simulink model "load_flow_analysis"  (R2014b)
settings: Solver=ode45  StartTime=0.0  StopTime=10.0  RelTol=1e-3
libraries: powerlib x13
settings Model: Creator=Amr Saleh  LastModifiedBy=Amr Saleh

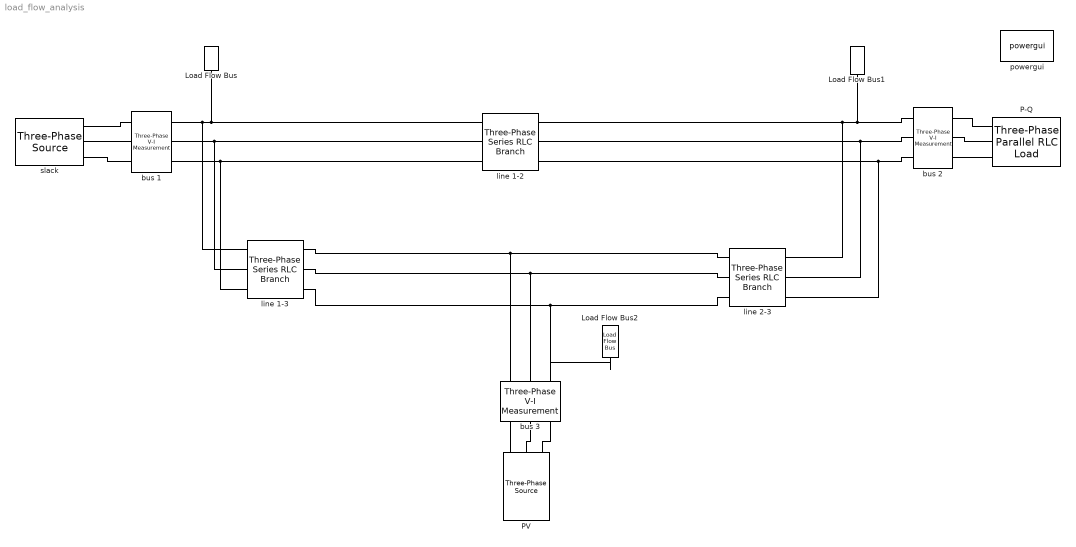
== system load_flow_analysis ==
  Load Flow Bus : powerlib/Measurements/Load Flow Bus  LConnTagsString=a  ID=BUS_1  Vbase=10e3  Vref=1.05  Vangle=0  VLF=1.05  angleLF=0
      settings: AttributesFormatString=%<ID>\n%<Vbase>V\n%<VLF>pu\n%<angleLF>deg.
  Load Flow Bus1 : powerlib/Measurements/Load Flow Bus  LConnTagsString=a  ID=BUS_2  Vbase=10e3  Vref=1  Vangle=0  VLF=0.9897  angleLF=1.546
      settings: AttributesFormatString=%<ID>\n%<Vbase>V\n%<VLF>pu\n%<angleLF>deg.
  Load Flow Bus2 : powerlib/Measurements/Load Flow Bus  LConnTagsString=a  ID=BUS_3  Vbase=10e3  Vref=1.04  Vangle=0  VLF=1.04  angleLF=3.427
      settings: AttributesFormatString=%<ID>\n%<Vbase>V\n%<VLF>pu\n%<angleLF>deg.
  P-Q : powerlib/Elements/Three-Phase Parallel RLC Load  LConnTagsString=A|B|C  Configuration=Y (grounded)  NominalVoltage=10e3  NominalFrequency=60  ActivePower=190e6  InductivePower=250e6  CapacitivePower=0  Measurements=None  LoadType=constant PQ
  PV : powerlib/Electrical Sources/Three-Phase Source  Voltage=10e3  PhaseAngle=0  Frequency=60  InternalConnection=Yg  SpecifyImpedance=off  Resistance=0.8929  Inductance=16.58e-3  ShortCircuitLevel=100e6  BaseVoltage=10e3  XRratio=7  BusType=PV  Pref=380e6  Qref=0  Qmin=-inf  Qmax=inf
  bus 1 : powerlib/Measurements/Three-Phase V-I Measurement  VoltageMeasurement=no  SetLabelV=off  LabelV=Vabc  Vpu=off  VpuLL=off  CurrentMeasurement=no  SetLabelI=off  LabelI=Iabc  Ipu=off  Pbase=100e6  Vbase=500e3  OutputType=Complex  PhasorSimulation=off  PSBequivalent=0
  bus 2 : powerlib/Measurements/Three-Phase V-I Measurement  VoltageMeasurement=no  SetLabelV=off  LabelV=Vabc  Vpu=off  VpuLL=off  CurrentMeasurement=no  SetLabelI=off  LabelI=Iabc  Ipu=off  Pbase=100e6  Vbase=500e3  OutputType=Complex  PhasorSimulation=off  PSBequivalent=0
  bus 3 : powerlib/Measurements/Three-Phase V-I Measurement  VoltageMeasurement=no  SetLabelV=off  LabelV=Vabc  Vpu=off  VpuLL=off  CurrentMeasurement=no  SetLabelI=off  LabelI=Iabc  Ipu=off  Pbase=100e6  Vbase=500e3  OutputType=Complex  PhasorSimulation=off  PSBequivalent=0
  line 1-2 : powerlib/Elements/Three-Phase Series RLC Branch  LConnTagsString=A|B|C  RConnTagsString=A|B|C  BranchType=RL  Resistance=0.02  Inductance=0.04/(2*pi*60)  Capacitance=1e-6  Measurements=None
  line 1-3 : powerlib/Elements/Three-Phase Series RLC Branch  LConnTagsString=A|B|C  RConnTagsString=A|B|C  BranchType=RL  Resistance=0.01  Inductance=0.03/(2*pi*60)  Capacitance=1e-6  Measurements=None
  line 2-3 : powerlib/Elements/Three-Phase Series RLC Branch  LConnTagsString=A|B|C  RConnTagsString=A|B|C  BranchType=RL  Resistance=0.0125  Inductance=0.025/(2*pi*60)  Capacitance=1e-6  Measurements=None
  powergui : powerlib/powergui  Priority=1  SimulationMode=Continuous  SolverType=Tustin/Backward Euler (TBE)  SampleTime=50e-6  frequency=60  SPID=off  DisableSnubberDevices=off  DisableRonSwitches=off  DisableVfSwitches=off  SwTol=0  DisplayEquations=off  Interpol=off  methode=off  Ts=100  frequencyindice=60  Pbase=100e6  ErrMax=0.0001  Iterations=50  UnitsV=kV  UnitsW=MW  FunctionMessages=off  echomessages=off  HookPort=off  EnableUseOfTLC=off  x0status=blocks  RestoreLinks=warning  ResistiveCurrentMeasurement=off  Frange=[0:2:500]  Ylog=off  Xlog=on  ShowGrid=off  save=off  variable=ZData  structure=0  ZoomFFT=off  StartTime=0.0  cycles=1  DisplayStyle=1  fundamental=60  FreqAxis=off  MaxFrequency=1000  frequencyindicesteady=1  RmsSteady=1  display=off
  slack : powerlib/Electrical Sources/Three-Phase Source  Voltage=10e3  PhaseAngle=0  Frequency=60  InternalConnection=Yg  SpecifyImpedance=off  Resistance=0.8929  Inductance=16.58e-3  ShortCircuitLevel=100e6  BaseVoltage=10e3  XRratio=7  BusType=swing  Pref=0  Qref=0  Qmin=-inf  Qmax=inf
  connections:
  slack/RConn1 -- bus 1/LConn1
  slack/RConn2 -- bus 1/LConn2
  slack/RConn3 -- bus 1/LConn3
  P-Q/LConn1 -- bus 2/RConn1
  P-Q/LConn2 -- bus 2/RConn2
  P-Q/LConn3 -- bus 2/RConn3
  bus 1/RConn1 -- line 1-2/LConn1 -- Load Flow Bus/LConn1 -- line 1-3/LConn1
  bus 1/RConn2 -- line 1-2/LConn2 -- line 1-3/LConn2
  line 1-2/LConn3 -- line 1-3/LConn3 -- bus 1/RConn3
  line 1-2/RConn1 -- line 2-3/RConn1 -- Load Flow Bus1/LConn1 -- bus 2/LConn1
  line 2-3/LConn2 -- bus 3/RConn2 -- line 1-3/RConn2
  line 2-3/LConn3 -- line 1-3/RConn3 -- Load Flow Bus2/LConn1 -- bus 3/RConn3
  PV/RConn1 -- bus 3/LConn1
  PV/RConn2 -- bus 3/LConn2
  PV/RConn3 -- bus 3/LConn3
  line 2-3/LConn1 -- bus 3/RConn1 -- line 1-3/RConn1
  line 1-2/RConn2 -- line 2-3/RConn2 -- bus 2/LConn2
  line 1-2/RConn3 -- line 2-3/RConn3 -- bus 2/LConn3
